simulink model "cheville"  (Simulink 7.8)
settings: Solver=ode45  StartTime=0.0  StopTime=2  RelTol=1e-3
libraries: simulink x3, slctrlblks x1
settings Model: Creator=Administrateur  LastModifiedBy=Administrateur
settings SolverCC: ZeroCrossAlgorithm=Adaptive

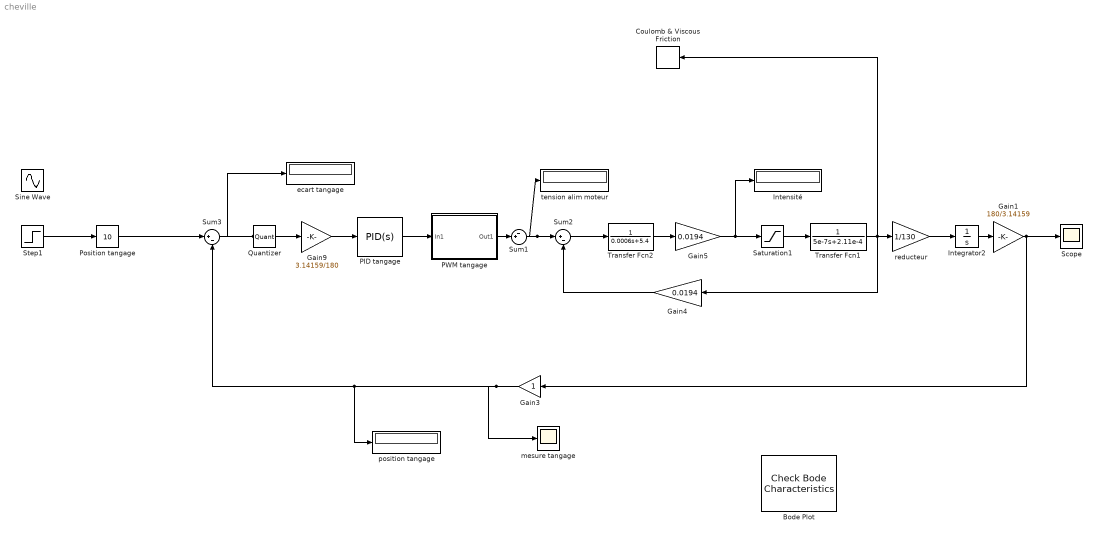
== system cheville ==
  Bode Plot : slctrlblks/Model Verification/Check Bode  Characteristics  LinearizationIOs={'/Position tangage', 1, 'in', 'on', '';'/Gain1', 1, 'out', 'on', ''}  LinearizeAt=SnapshotTimes  SnapshotTimes=[0]  TriggerType=rising  SampleTime=auto  RateConversionMethod=zoh  PreWarpFreq=10  UseExactDelayModel=off  UseFullBlockNameLabels=off  UseBusSignalLabels=off  enabled=on  stopWhenAssertionFail=off  export=off  ViewDlgPos=[100 200 510 390]  OpenViewOnLoad=off  LaunchViewOnOpen=off  FrequencyUnits=rad/s  MagnitudeUnits=dB  PhaseUnits=deg  TimeUnits=seconds  EnableUpperBound=off  UpperBoundFrequencies=[]  UpperBoundMagnitudes=[]  EnableLowerBound=off  LowerBoundFrequencies=[]  LowerBoundMagnitudes=[]
  Coulomb & Viscous Friction : simulink/Discontinuities/Coulomb & Viscous Friction  offset=0.01  gain=1
  Gain1 : Gain  Gain=180/3.14159
  Gain3 : Gain
  Gain4 : Gain  Gain=0.0194
  Gain5 : Gain  Gain=0.0194
  Gain9 : Gain  Gain=3.14159/180
  Integrator2 : Integrator
  Intensité : Display
  PID tangage : simulink/Continuous/PID Controller  Controller=PID  TimeDomain=Continuous-time  SampleTime=1  IntegratorMethod=Forward Euler  FilterMethod=Forward Euler  Form=Parallel  P=1500  I=0  D=0  N=100  InitialConditionSource=internal  InitialConditionForIntegrator=0  InitialConditionForFilter=0  ExternalReset=none  LimitOutput=off  UpperSaturationLimit=inf  LowerSaturationLimit=-inf  LinearizeAsGain=off  AntiWindupMode=none  Kb=1  TrackingMode=off  Kt=1  PParamMin=[]  PParamMax=[]  IParamMin=[]  IParamMax=[]  DParamMin=[]  DParamMax=[]  NParamMin=[]  NParamMax=[]  KbParamMin=[]  KbParamMax=[]  KtParamMin=[]  KtParamMax=[]  POutMin=[]  POutMax=[]  IOutMin=[]  IOutMax=[]  DOutMin=[]  DOutMax=[]  NOutMin=[]  NOutMax=[]  KbOutMin=[]  KbOutMax=[]  KtOutMin=[]  KtOutMax=[]  IntegratorOutMin=[]  IntegratorOutMax=[]  FilterOutMin=[]  FilterOutMax=[]  SumOutMin=[]  SumOutMax=[]  SumI1OutMin=[]  SumI1OutMax=[]  SumI2OutMin=[]  SumI2OutMax=[]  SumI3OutMin=[]  SumI3OutMax=[]  SumDOutMin=[]  SumDOutMax=[]  SaturationOutMin=[]  SaturationOutMax=[]  IntegratorContinuousStateAttributes=''  IntegratorStateMustResolveToSignalObject=off  IntegratorRTWStateStorageClass=Auto  FilterContinuousStateAttributes=''  FilterStateMustResolveToSignalObject=off  FilterRTWStateStorageClass=Auto
  PWM tangage : Subsystem
  Position tangage : simulink/Math Operations/Slider Gain  low=-180  gain=10  high=180
  Quantizer : Quantizer  QuantizationInterval=4e-3
  Saturation1 : Saturate  UpperLimit=0.068  LowerLimit=-0.068
  Scope : Scope
      settings: YMin=0  YMax=10
  Sine Wave : Sin  Frequency=10  SampleTime=0
  Step1 : Step  Time=1e-7  SampleTime=0
  Sum1 : Sum  Inputs=-+|
  Sum2 : Sum  Inputs=|+-
  Sum3 : Sum  Inputs=|+-
  Transfer Fcn1 : TransferFcn  Denominator=[5e-7 2.11e-4]
  Transfer Fcn2 : TransferFcn  Denominator=[0.0006 5.4]
  ecart tangage : Display
  mesure tangage : Scope
      settings: TimeRange=0.3  YMin=-0.75  YMax=2
  position tangage : Display
  reducteur : Gain  Gain=1/130
  tension alim moteur : Display
  wires:
  Transfer Fcn2/1 -> Gain5/1
  Sum2/1 -> Transfer Fcn2/1
  Sum3/1 -> ecart tangage/1, Quantizer/1
  PID tangage/1 -> PWM tangage/1(In1)
  Gain4/1 -> Sum2/2
  Gain5/1 -> Saturation1/1, Intensité/1
  Position tangage/1 -> Sum3/1
  Gain3/1 -> mesure tangage/1, Sum3/2, position tangage/1
  Gain9/1 -> PID tangage/1
  Saturation1/1 -> Transfer Fcn1/1
  Transfer Fcn1/1 -> reducteur/1, Gain4/1, Coulomb & Viscous Friction/1
  reducteur/1 -> Integrator2/1
  Integrator2/1 -> Gain1/1
  Gain1/1 -> Scope/1, Gain3/1
  Quantizer/1 -> Gain9/1
  Step1/1 -> Position tangage/1
  PWM tangage/1(Out1) -> Sum1/2
  Sum1/1 -> Sum2/1, tension alim moteur/1

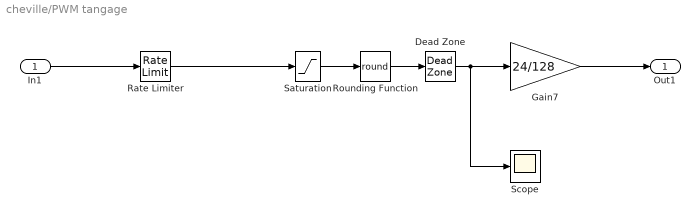
== system cheville/PWM tangage ==
  In1 : Inport
  Dead Zone : DeadZone  LowerValue=-1  UpperValue=1  SaturateOnIntegerOverflow=on
  Gain7 : Gain  Gain=24/128
  Rate Limiter : RateLimiter  RisingSlewLimit=5000  FallingSlewLimit=-5000  SampleTimeMode=inherited
  Rounding Function : Rounding  Operator=round
  Saturation : Saturate  UpperLimit=128  LowerLimit=-128
  Scope : Scope
      settings: YMin=68  YMax=68  SaveName=ScopeData2
  Out1 : Outport
  wires:
  Rounding Function/1 -> Dead Zone/1
  Saturation/1 -> Rounding Function/1
  Dead Zone/1 -> Gain7/1, Scope/1
  Gain7/1 -> Out1/1
  In1/1 -> Rate Limiter/1
  Rate Limiter/1 -> Saturation/1
